simulink model "mpc_blendingprocess"  (R2023a)
settings: Solver=ode45  StartTime=0.0  StopTime=16  RelTol=1e-3  EnableMultiTasking=on
libraries: mpclib x1
settings Model: Creator=The MathWorks, Inc.  LastModifiedBy=The MathWorks, Inc.
settings SolverCC: AlgebraicLoopSolver=TrustRegion  MaxZcPerStep=1
settings DataIOCC: LimitDataPoints=on  SaveFormat=Array  ReturnWorkspaceOutputs=off
settings OptimizationCC: ReuseModelBlockBuffer=off  ExpressionDepthLimit=2147483647  LifeSpan=inf
settings DebuggingCC: UnderspecifiedInitializationDetection=Classic  MergeDetectMultiDrivingBlocksExec=none  FcnCallInpInsideContextMsg=warning  UnconnectedInputMsg=warning  UnconnectedOutputMsg=warning  UnconnectedLineMsg=warning  StateNameClashWarn=warning  SFUnexpectedBacktrackingDiag=warning  SFNoUnconditionalDefaultTransitionDiag=warning  SFExecutionAtInitializationDiag=none  ArithmeticOperatorsInVariantConditions=warning
settings HardwareCC: ProdBitPerPointer=32  ProdBitPerSizeT=32  ProdBitPerPtrDiffT=32  ProdLargestAtomicFloat=None  ProdIntDivRoundTo=Undefined  ProdEndianess=Unspecified  ProdWordSize=32  ProdHWDeviceType=32-bit Generic
settings ModelReferenceCC: EnableRefExpFcnMdlSchedulingChecks=on  PropagateSignalLabelsOutOfModel=off
settings SFSimCC: SimUseLocalCustomCode=off  CustomCodeUndefinedFunction=UseInterfaceOnly
settings RTWCC: RTWUseLocalCustomCode=off  DLArmComputeVersion=19.05
settings CodeAppCC: StateflowObjectComments=on
settings GRTTargetCC: TargetLangStandard=C89/C90 (ANSI)  CombineOutputUpdateFcns=off  GRTInterface=on
settings ConfigComp: CovMetricSettings=dw  CovSaveCumulativeToWorkspaceVar=on  CovSaveSingleToWorkspaceVar=on  CovExternalEMLEnable=off  CovSFcnEnable=off

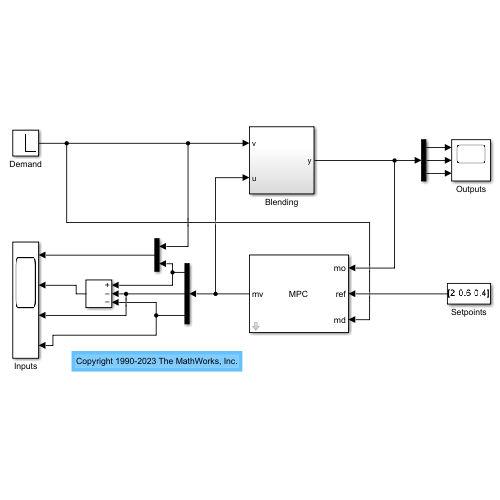
[thumbnail: Simulink's stored preview of the top-level diagram]
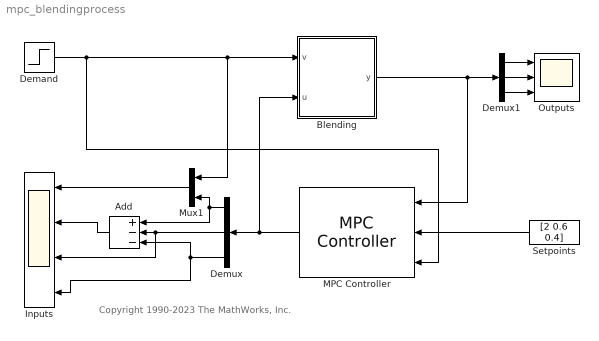
== system mpc_blendingprocess ==
  note: Copyright 1990-2023 The MathWorks, Inc.
  Add : Sum  Inputs=+--
  Blending : Subsystem
  Demand : Step  Before=2  After=1.8  SampleTime=0
  Demux : Demux  Outputs=3
  Demux1 : Demux  Outputs=3
  Inputs : Scope  NumInputPorts=4
  MPC Controller : mpclib/MPC Controller  mpcobj=mpcobj  x0=[]  is_multiple=0  enable_value=0  return_u0=off  updateMPCinCallerWorkspace=on  md_inport=on  mv_inport=off  uref_inport=off  return_cost=off  return_mvseq=off  return_qpstatus=off  return_xseq=off  return_state=off  return_ovseq=off  state_inport=off  umin_inport=off  umax_inport=off  ymin_inport=off  ymax_inport=off  cc_inport=off  ywt_inport=off  uwt_inport=off  duwt_inport=off  rhoeps_inport=off  pm_inport=off  MaximumP=10  HorizonChoice=FixedHorizon  n_ts=0.1  n_p=10  n_mv=3  n_md=1  n_ud=0  n_mo=3  n_uo=0  BlockDataType=double  SampleTimeInherited=off  switch_inport=off
  Mux1 : Mux  Inputs=2
  Outputs : Scope  NumInputPorts=3
  Setpoints : Constant  Value=[2 0.6 0.4]
  wires:
  Demux1/3 -> Outputs/3
  Demux1/2 -> Outputs/2
  Demux1/1 -> Outputs/1
  Demux/2 -> Add/2, Inputs/3
  Demux/3 -> Inputs/4, Add/3
  Mux1/1 -> Inputs/1
  Demux/1 -> Add/1, Mux1/2
  Demand/1 -> Mux1/1, Blending/1(v), MPC Controller/3
  Setpoints/1 -> MPC Controller/2
  MPC Controller/1 -> Blending/2(u), Demux/1
  Blending/1(y) -> MPC Controller/1, Demux1/1
  Add/1 -> Inputs/2

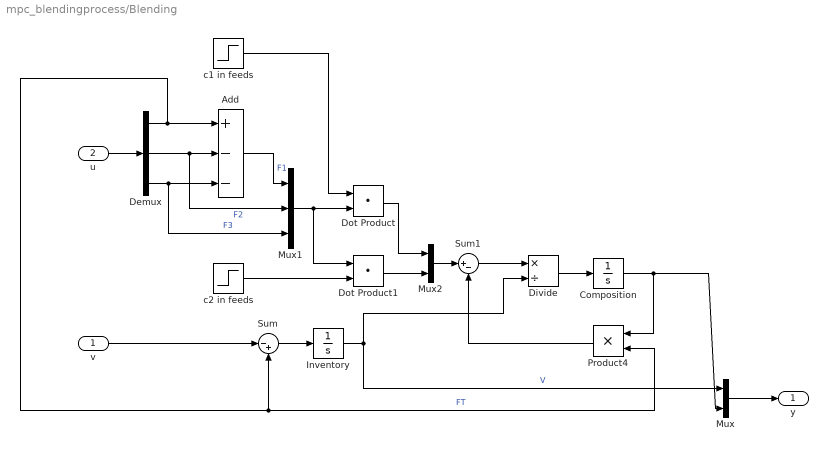
== system mpc_blendingprocess/Blending ==
  v : Inport
  u : Inport  Port=2
  Add : Sum  Inputs=+--
  Composition : Integrator  InitialCondition=[0.6 0.4]  LimitOutput=on  LowerSaturationLimit=0
  Demux : Demux  Outputs=3
  Divide : Product  Inputs=*/
  Dot Product : DotProduct  OutDataTypeStr=Inherit: Inherit via internal rule
  Dot Product1 : DotProduct  OutDataTypeStr=Inherit: Inherit via internal rule
  Inventory : Integrator  InitialCondition=2  LimitOutput=on  LowerSaturationLimit=1e-5
  Mux : Mux  Inputs=2
  Mux1 : Mux  Inputs=3
  Mux2 : Mux  Inputs=2
  Product4 : Product  RndMeth=Zero
  Sum : Sum  Inputs=|-+
  Sum1 : Sum  Inputs=|+-
  c1 in feeds : Step  Time=2  Before=[0.7 0.2 0.5]  After=[0.6 0.2 0.4]  SampleTime=0
  c2 in feeds : Step  Time=2  Before=[0.3 0.8 0.4]  After=[0.4 0.8 0.4]  SampleTime=0
  y : Outport
  wires:
  Add/1 -> Mux1/1  "F1"
  Mux1/1 -> Dot Product/2, Dot Product1/1
  Demux/3 -> Mux1/3, Add/3  "F3"
  Demux/2 -> Mux1/2, Add/2  "F2"
  Demux/1 -> Add/1, Product4/2, Sum/2  "FT"
  u/1 -> Demux/1
  v/1 -> Sum/1
  Mux/1 -> y/1
  Product4/1 -> Sum1/2
  Divide/1 -> Composition/1
  Sum1/1 -> Divide/1
  Composition/1 -> Mux/2, Product4/1
  Inventory/1 -> Divide/2, Mux/1  "V"
  Sum/1 -> Inventory/1
  Mux2/1 -> Sum1/1
  c1 in feeds/1 -> Dot Product/1
  Dot Product/1 -> Mux2/1
  Dot Product1/1 -> Mux2/2
  c2 in feeds/1 -> Dot Product1/2
